simulink library "FirUp"  (R2022b)
settings: Solver=VariableStepAuto  StartTime=0.0  StopTime=10.0  RelTol=1e-3
undefined symbols (not defined in the file or in its folder): Row
libraries: HandyTextFile x10, FeaturePath x2, ITC x2, $bdroot x2, TuneVar x2, dspmlti4 x1, FirGeneric x1, TOP x1
settings Model: Creator=jb10849  LastModifiedBy=sc48041
settings SolverCC: AlgebraicLoopSolver=TrustRegion
settings DebuggingCC: UnconnectedInputMsg=warning  UnconnectedOutputMsg=warning  UnconnectedLineMsg=warning  SFMachineParentedDataDiag=warning  ArithmeticOperatorsInVariantConditions=warning
settings ModelReferenceCC: EnableRefExpFcnMdlSchedulingChecks=on
settings SFSimCC: SimUseLocalCustomCode=off  CustomCodeUndefinedFunction=UseInterfaceOnly
settings RTWCC: RTWUseLocalCustomCode=off  DLArmComputeVersion=19.05
settings CodeAppCC: StateflowObjectComments=on

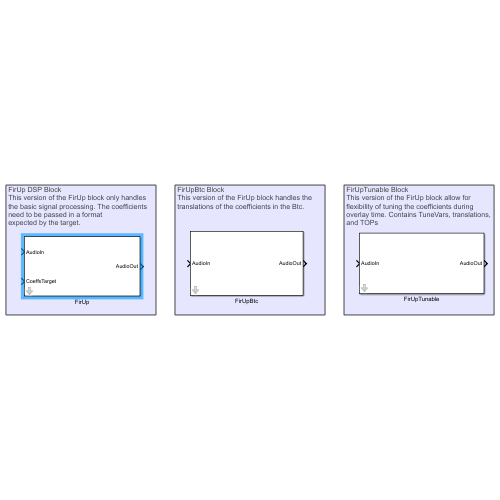
[thumbnail: Simulink's stored preview of the top-level diagram]
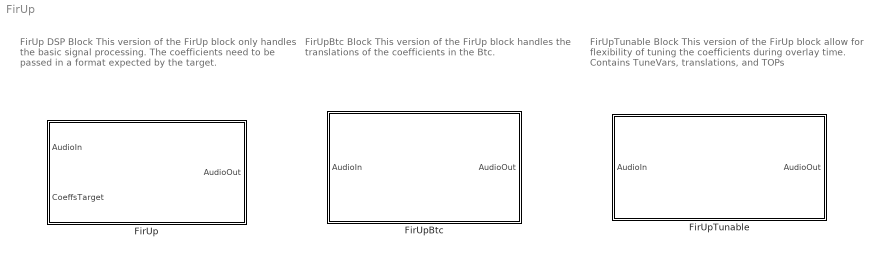
== system FirUp ==
  note: FirUp DSP Block
      | This version of the FirUp block only handles
      | the basic signal processing. The coefficients
      | need to be passed in a format
      | expected by the target.
  note: FirUpBtc Block
      | This version of the FirUp block handles the
      | translations of the coefficients in the Btc.
  note: FirUpTunable Block
      | This version of the FirUp block allow for
      | flexibility of tuning the coefficients during
      | overlay time. Contains TuneVars, translations,
      | and TOPs
  FirUp : Subsystem  mask(Blocklib FirUp){Config=[]}
      mask prompts: Config "FirUpConfig"
      mask init:
      | blkh=gcbh;
      | Config=BTConfig.Assert(blkh,Config);
      | 
      | Config.Validate();
      | Config.DoMaskInit(blkh);
      mask DialogControl ParamterGroupVar Prompt: Parameters
  FirUpBtc : Subsystem  mask(Blocklib FirUpBtc){Config=[]}
      mask prompts: Config "FirUpBtcConfig"
      mask init:
      | blkh=gcbh;
      | Config=BTConfig.Assert(blkh,Config);
      | 
      | Config.Validate();
      | Config.DoMaskInit(blkh);
  FirUpTunable : Subsystem  mask(Blocklib FirUpTunable){Config=[]}
      mask prompts: Config "FirUpTunableConfig"
      mask init:
      | blkh=gcbh;
      | Config=BTConfig.Assert(blkh,Config);
      | 
      | Config.Validate();
      | Config.DoMaskInit(blkh);

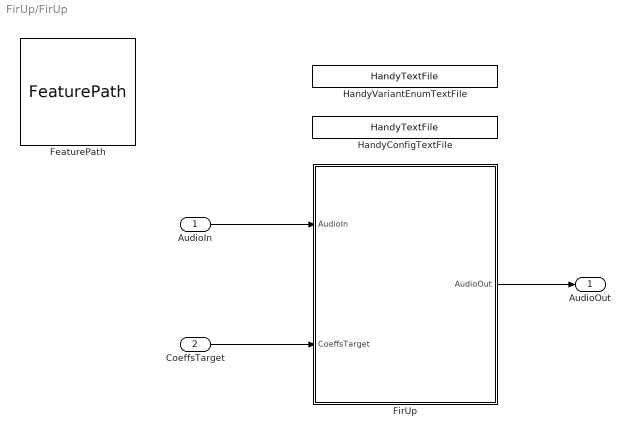
== system FirUp/FirUp ==
  AudioIn : Inport
  CoeffsTarget : Inport  Port=2
  FeaturePath : FeaturePath/FeaturePath  FeatureName=FirUp  IsGroup=off  GroupNumber=-1  IsModule=off  TriggerInit=[125 24 240 131]
      settings: SourceProductName=Bose Talaria
  FirUp : Subsystem  Variant=on
  HandyConfigTextFile : HandyTextFile/HandyTextFile  TemplateSource=Config  FileSuffix=File  OpenDialogOnLoad=off  UseThisBlockName=off  AddGrandParentNamePrefix=off  TheDefaultText=% $(FILENAME) $(PREFIX) $(SUFFIX)  ShowInLibBrowser=on
      settings: SourceProductName=Bose Talaria
  HandyVariantEnumTextFile : HandyTextFile/HandyTextFile  TemplateSource=VariantEnum  FileSuffix=File  OpenDialogOnLoad=off  UseThisBlockName=off  AddGrandParentNamePrefix=off  TheDefaultText=% $(FILENAME) $(PREFIX) $(SUFFIX)  ShowInLibBrowser=on
      settings: SourceProductName=Bose Talaria
  AudioOut : Outport
  wires:
  FirUp/1(AudioOut) -> AudioOut/1
  CoeffsTarget/1 -> FirUp/2(CoeffsTarget)
  AudioIn/1 -> FirUp/1(AudioIn)

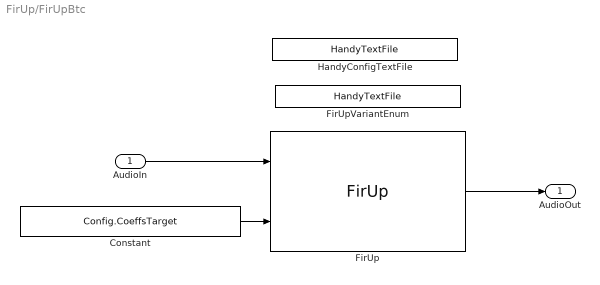
== system FirUp/FirUpBtc ==
  AudioIn : Inport
  Constant : Constant  Value=Config.CoeffsTarget  VectorParams1D=off  OutDataTypeStr=single
  FirUp : $bdroot/FirUp  Config=Config
  FirUpVariantEnum : HandyTextFile/HandyTextFile  TemplateSource=<dialog fields>  FileSuffix=VariantEnum  OpenDialogOnLoad=off  UseThisBlockName=on  AddGrandParentNamePrefix=off  TheDefaultText=% $(FILENAME) $(PREFIX) $(SUFFIX)  ShowInLibBrowser=on
      settings: SourceProductName=Bose Talaria
  HandyConfigTextFile : HandyTextFile/HandyTextFile  TemplateSource=Config  FileSuffix=File  OpenDialogOnLoad=off  UseThisBlockName=off  AddGrandParentNamePrefix=off  TheDefaultText=% $(FILENAME) $(PREFIX) $(SUFFIX)  ShowInLibBrowser=on
      settings: SourceProductName=Bose Talaria
  AudioOut : Outport
  wires:
  AudioIn/1 -> FirUp/1
  FirUp/1 -> AudioOut/1
  Constant/1 -> FirUp/2

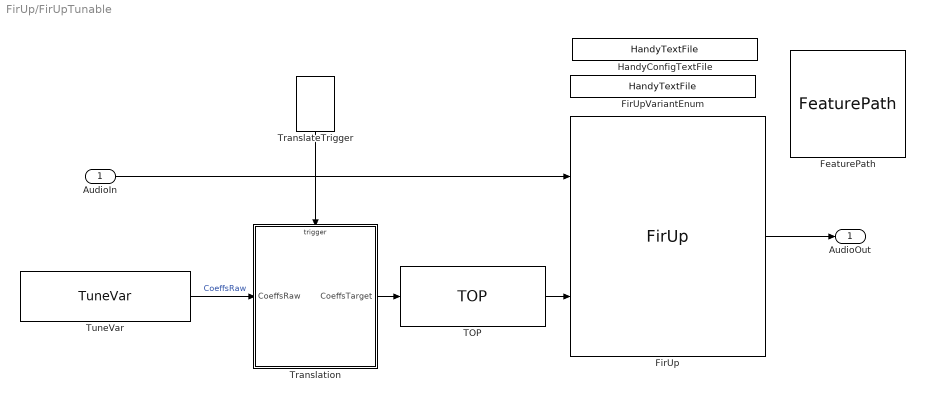
== system FirUp/FirUpTunable ==
  AudioIn : Inport
  FeaturePath : FeaturePath/FeaturePath  FeatureName=FirUp  IsGroup=off  GroupNumber=-1  IsModule=off  TriggerInit=[415 9 530 116]
      settings: SourceProductName=Bose Talaria
  FirUp : $bdroot/FirUp  Config=Config
  FirUpVariantEnum : HandyTextFile/HandyTextFile  TemplateSource=<dialog fields>  FileSuffix=File  OpenDialogOnLoad=off  UseThisBlockName=off  AddGrandParentNamePrefix=off  TheDefaultText=% $(FILENAME) $(PREFIX) $(SUFFIX)  ShowInLibBrowser=on
      settings: SourceProductName=Bose Talaria
  HandyConfigTextFile : HandyTextFile/HandyTextFile  TemplateSource=Config  FileSuffix=File  OpenDialogOnLoad=off  UseThisBlockName=off  AddGrandParentNamePrefix=off  TheDefaultText=% $(FILENAME) $(PREFIX) $(SUFFIX)  ShowInLibBrowser=on
      settings: SourceProductName=Bose Talaria
  TOP : TOP/TOP  TriggerInit=[25 225 170 285]  TopName=CoeffsTarget  DataTypeOut=Inherit: Same as input  BankNumber=0  PreOverlay=false  PostOverlay=false  Role=Automatic
      settings: SourceProductName=Bose Talaria
  TranslateTrigger : TuneVar/TranslateTrigger  TriggerInit=[-79 35 -41 90]
      settings: SourceProductName=Bose Talaria
  Translation : MATLAB Function  TreatAsAtomicUnit=on  mask(Talaria Translation){UpFactor=Config.UpFactor, VariantStr=Config.Variant.Uint8Str, WithFirVariantStr=Config.WithFirVariant.Uint8Str}
      mask help: This MATLAB Function Block can be automatically inserted by several automation routines. Once placed, the block is ready to accept translation logic from the model designer.
  TuneVar : TuneVar/TuneVar  TuneName=CoeffsRaw  SpecifyMaxSize=off  VariableDim=1 (Row)  MaxSize=[1 1]  TunabilityNumber=1  MinValue=[]  MaxValue=[]  TriggerInit=[-355 230 -185 280]  MaskValue=Config.TuneVarCoeffsRaw
      settings: SourceProductName=Bose Talaria
  AudioOut : Outport
  wires:
  FirUp/1 -> AudioOut/1
  AudioIn/1 -> FirUp/1
  TranslateTrigger/1 -> Translation/Trigger
  TuneVar/1 -> Translation/1(CoeffsRaw)  "CoeffsRaw"
  Translation/1(CoeffsTarget) -> TOP/1
  TOP/1 -> FirUp/2

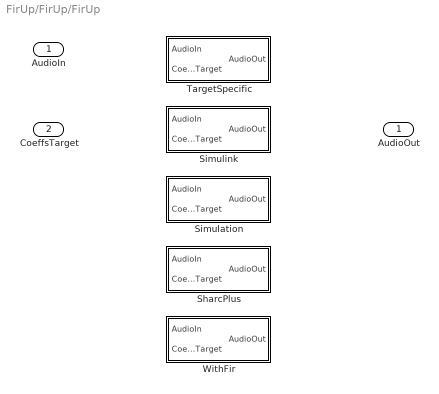
== system FirUp/FirUp/FirUp ==
  AudioIn : Inport
  CoeffsTarget : Inport  Port=2
  SharcPlus : Subsystem  VariantControl=Config.Variant.StartsWith('SharcPlus')
  Simulation : Subsystem  VariantControl=Config.Variant.StartsWith('Simulation')
  Simulink : Subsystem  VariantControl=(default)
  TargetSpecific : Subsystem  VariantControl=Config.Variant.StartsWith('Generic') || Config.Variant.StartsWith('Hexagon')
  WithFir : Subsystem  VariantControl=Config.Variant.StartsWith('WithFir')
  AudioOut : Outport

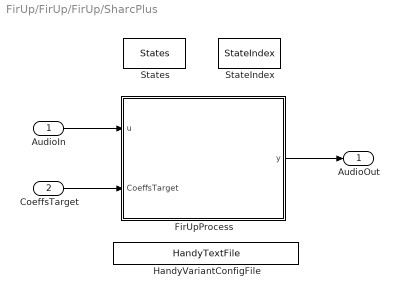
== system FirUp/FirUp/FirUp/SharcPlus ==
  AudioIn : Inport
  CoeffsTarget : Inport  Port=2
  FirUpProcess : MATLAB Function  TreatAsAtomicUnit=on  mask{UpFactor=Config.UpFactor}
  HandyVariantConfigFile : HandyTextFile/HandyTextFile  TemplateSource=VariantConfig  FileSuffix=Init  OpenDialogOnLoad=off  UseThisBlockName=off  AddGrandParentNamePrefix=on  TheDefaultText=|  ShowInLibBrowser=on
      | % $(FILENAME) Setup model parameters for each "Init" callback (e.g. update diagram)
      | sample_rate_in_hertz = 44100;
      | frame_size = 32;
      | sysin_channel_count = 2;
      settings: SourceProductName=Bose Talaria
  StateIndex : DataStoreMemory  DataStoreName=StateIndex  InitialValue=Config.VariantObj.DsmStateIndexInitValue  ShowAdditionalParam=off  OutDataTypeStr=int32
  States : DataStoreMemory  DataStoreName=States  InitialValue=Config.VariantObj.DsmStatesInitValue  ShowAdditionalParam=off  OutDataTypeStr=single
  AudioOut : Outport
  wires:
  FirUpProcess/1(y) -> AudioOut/1
  AudioIn/1 -> FirUpProcess/1(u)
  CoeffsTarget/1 -> FirUpProcess/2(CoeffsTarget)

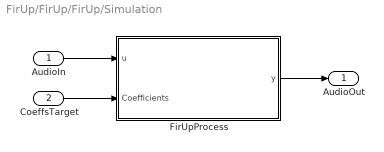
== system FirUp/FirUp/FirUp/Simulation ==
  AudioIn : Inport
  CoeffsTarget : Inport  Port=2
  FirUpProcess : MATLAB Function  TreatAsAtomicUnit=on  mask{UpFactor=Config.UpFactor}
  AudioOut : Outport
  wires:
  AudioIn/1 -> FirUpProcess/1(u)
  FirUpProcess/1(y) -> AudioOut/1
  CoeffsTarget/1 -> FirUpProcess/2(Coefficients)

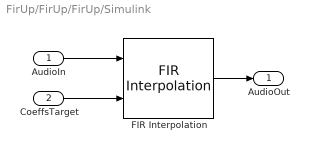
== system FirUp/FirUp/FirUp/Simulink ==
  AudioIn : Inport  OutDataTypeStr=single
  CoeffsTarget : Inport  Port=2  OutDataTypeStr=single
  FIR Interpolation : dspmlti4/FIR Interpolation  FilterSource=Input port  PrivateCoeffs=0  h=Config.Coefficients  L=Config.UpFactor  FilterObject=FINTERP  InputProcessing=Columns as channels (frame based)  framing=Enforce single-rate processing  outputBufInitCond=0  roundingMode=Floor  overflowMode=off  firstCoeffDataTypeStr=Inherit: Same word length as input  firstCoeffMin=[]  firstCoeffMax=[]  firstCoeffLastDataTypeStr=Inherit: Same word length as input  outputDataTypeStr=Inherit: Same as accumulator  outputMin=[]  outputMax=[]  outputLastDataTypeStr=Inherit: Same as accumulator
  AudioOut : Outport  OutDataTypeStr=single
  wires:
  AudioIn/1 -> FIR Interpolation/1
  FIR Interpolation/1 -> AudioOut/1
  CoeffsTarget/1 -> FIR Interpolation/2

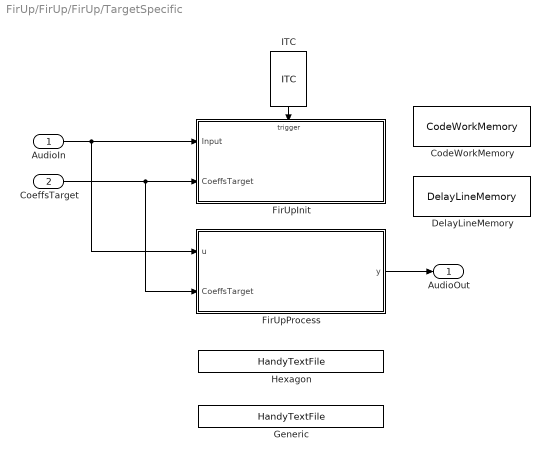
== system FirUp/FirUp/FirUp/TargetSpecific ==
  AudioIn : Inport
  CoeffsTarget : Inport  Port=2
  CodeWorkMemory : DataStoreMemory  DataStoreName=CodeWorkMemory  WriteAfterWriteMsg=warning  InitialValue=Config.VariantObj.CodeWorkMemoryInitValue  ShowAdditionalParam=off  OutDataTypeStr=uint32
  DelayLineMemory : DataStoreMemory  DataStoreName=DelayLineMemory  WriteAfterWriteMsg=warning  InitialValue=Config.VariantObj.DelayLineMemoryInitValue  ShowAdditionalParam=off  OutDataTypeStr=single
  FirUpInit : MATLAB Function  TreatAsAtomicUnit=on  mask{UpFactor=Config.UpFactor, VariantUint8=Config.Variant.Uint8Str}
  FirUpProcess : MATLAB Function  TreatAsAtomicUnit=on  mask{UpFactor=Config.UpFactor, VariantUint8=Config.Variant.Uint8Str}
  Generic : HandyTextFile/HandyTextFile  TemplateSource=VariantConfig  FileSuffix=Init  OpenDialogOnLoad=off  UseThisBlockName=on  AddGrandParentNamePrefix=on  TheDefaultText=|  ShowInLibBrowser=on
      | % $(FILENAME) Setup model parameters for each "Init" callback (e.g. update diagram)
      | sample_rate_in_hertz = 44100;
      | frame_size = 32;
      | sysin_channel_count = 2;
      settings: SourceProductName=Bose Talaria
  Hexagon : HandyTextFile/HandyTextFile  TemplateSource=VariantConfig  FileSuffix=Init  OpenDialogOnLoad=off  UseThisBlockName=on  AddGrandParentNamePrefix=on  TheDefaultText=|  ShowInLibBrowser=on
      | % $(FILENAME) Setup model parameters for each "Init" callback (e.g. update diagram)
      | sample_rate_in_hertz = 44100;
      | frame_size = 32;
      | sysin_channel_count = 2;
      settings: SourceProductName=Bose Talaria
  ITC : ITC/ITC
      settings: SourceProductName=Bose Talaria
  AudioOut : Outport
  wires:
  FirUpProcess/1(y) -> AudioOut/1
  ITC/1 -> FirUpInit/Trigger
  AudioIn/1 -> FirUpProcess/1(u), FirUpInit/1(Input)
  CoeffsTarget/1 -> FirUpProcess/2(CoeffsTarget), FirUpInit/2(CoeffsTarget)

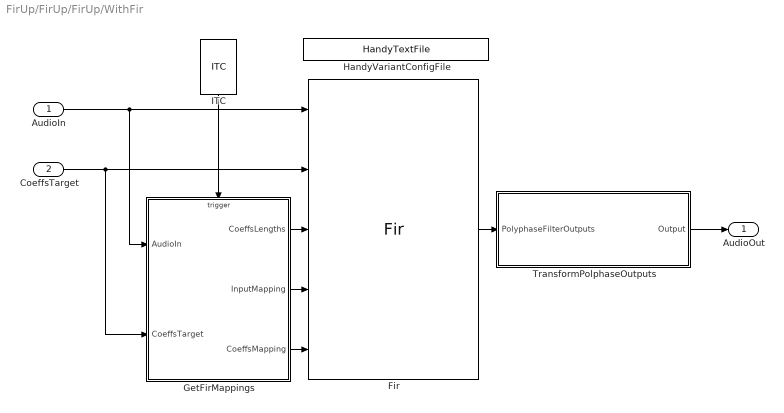
== system FirUp/FirUp/FirUp/WithFir ==
  AudioIn : Inport
  CoeffsTarget : Inport  Port=2
  Fir : FirGeneric/Fir  Config=Config.VariantObj.Fir
      settings: SourceProductName=Bose Blocklib
  GetFirMappings : MATLAB Function  TreatAsAtomicUnit=on  mask{UpFactor=Config.UpFactor}
  HandyVariantConfigFile : HandyTextFile/HandyTextFile  TemplateSource=VariantConfig  FileSuffix=Init  OpenDialogOnLoad=off  UseThisBlockName=off  AddGrandParentNamePrefix=on  TheDefaultText=|  ShowInLibBrowser=on
      | % $(FILENAME) Setup model parameters for each "Init" callback (e.g. update diagram)
      | sample_rate_in_hertz = 44100;
      | frame_size = 32;
      | sysin_channel_count = 2;
      settings: SourceProductName=Bose Talaria
  ITC : ITC/ITC
      settings: SourceProductName=Bose Talaria
  TransformPolphaseOutputs : MATLAB Function  TreatAsAtomicUnit=on  mask{UpFactor=Config.UpFactor}
  AudioOut : Outport
  wires:
  GetFirMappings/1(CoeffsLengths) -> Fir/3
  GetFirMappings/3(CoeffsMapping) -> Fir/5
  GetFirMappings/2(InputMapping) -> Fir/4
  ITC/1 -> GetFirMappings/Trigger
  TransformPolphaseOutputs/1(Output) -> AudioOut/1
  CoeffsTarget/1 -> GetFirMappings/2(CoeffsTarget), Fir/2
  Fir/1 -> TransformPolphaseOutputs/1(PolyphaseFilterOutputs)
  AudioIn/1 -> GetFirMappings/1(AudioIn), Fir/1

== matlab function FirUp/FirUp/TargetSpecific/FirUpProcess ==
  data: u input; y output; UpFactor parameter; DelayLineMemory data_store_memory; CodeWorkMemory data_store_memory; VariantUint8 parameter; CoeffsTarget input
function y = FirUpProcess(u, UpFactor, VariantUint8, CoeffsTarget)
% Upsample the input signal by an integer-valued factor, then apply an 
% FIR filter. 

global DelayLineMemory;
global CodeWorkMemory;
VariantSelect = char(VariantUint8);

if(coder.target('MATLAB') || coder.target('Sfun')) 
    y = FirUpProcessSim(u, CoeffsTarget, UpFactor, VariantSelect);
else
    switch(VariantSelect)
        case('Generic')
            y = firup_generic_process(single(u), single(DelayLineMemory), uint32(CodeWorkMemory), uint32(UpFactor));
        case('Hexagon')
            y = firup_hexagon_process(single(u), single(DelayLineMemory), uint32(CodeWorkMemory), uint32(UpFactor));
    end
end
end

function y = firup_generic_process(u, DelayLineMemory, CodeWorkMemory, UpFactor)
coder.replace('-errorifnoreplacement');
[FrameSize, NumChannels] = size(u);
y = single(zeros(FrameSize*UpFactor, NumChannels));
end
function y = firup_hexagon_process(u, DelayLineMemory, CodeWorkMemory, UpFactor)
coder.replace('-errorifnoreplacement');
[FrameSize, NumChannels] = size(u);
y = single(zeros(FrameSize*UpFactor, NumChannels));
end

== matlab function FirUp/FirUp/SharcPlus/FirUpProcess ==
  data: u input; CoeffsTarget input; y output; UpFactor parameter; States data_store_memory; StateIndex data_store_memory
function y = FirUpProcess(u, CoeffsTarget, UpFactor)
% Upsample the input signal by an integer-valued factor, then apply an 
% FIR filter. 
global States;
global StateIndex;

if(coder.target('MATLAB') || coder.target('Sfun')) 
    y = FirUpProcessSim(u, CoeffsTarget, UpFactor, "SharcPlus");
else
    [FrameSize, NumChannels] = size(u);
    ActiveCoeffSet = zeros(NumChannels,1);
    PolyphaseFilterLength = numel(CoeffsTarget)/ UpFactor;
    y = upfir(single(u), uint32(FrameSize*UpFactor), uint32(NumChannels), single(States), ...
        int32(numel(CoeffsTarget)), int32(StateIndex), single(CoeffsTarget), ...
        uint32(ActiveCoeffSet), int32(UpFactor), int32(PolyphaseFilterLength));
end
end

function y = upfir(u, framesize, numChannels, states2, filterLength, stateIndex2, coeffs, activeCoeffSet, interp_factor, polylen)
% If target == codegen, generate warning if no CRL found
coder.replace('-errorifnoreplacement');
y = single(zeros(framesize , numChannels));
end

== matlab function FirUp/FirUp/TargetSpecific/FirUpInit ==
  data: Input input; UpFactor parameter; CodeWorkMemory data_store_memory; VariantUint8 parameter; CoeffsTarget input
  events: trigger input FUNCTION_CALL_EVENT
function FirUpInit(Input, UpFactor, VariantUint8, CoeffsTarget)

global CodeWorkMemory;

VariantSelect = char(VariantUint8);
[FrameSize, NumChannels] = size(Input);
FilterLength = numel(CoeffsTarget);
if(coder.target('MATLAB') || coder.target('Sfun')) 
    return;
else
    switch(VariantSelect)
        case('Generic')
            y = firup_generic_init(single(CoeffsTarget), uint32(FrameSize), uint32(UpFactor), uint32(FilterLength), uint32(NumChannels), uint32(CodeWorkMemory));
            % NOTE: The CRL mechanism requires an output for the function call,
            % and appears to be optimized out if that return value isn't used. 
            % This is a dummy operation to make sure CRL ends up in generated code
            CodeWorkMemory(1) = y;
        case('Hexagon')
            y = firup_hexagon_init(single(CoeffsTarget), uint32(FrameSize), uint32(UpFactor), uint32(FilterLength), uint32(NumChannels), uint32(CodeWorkMemory));
            % NOTE: The CRL mechanism requires an output for the function call,
            % and appears to be optimized out if that return value isn't used. 
            % This is a dummy operation to make sure CRL ends up in generated code
            CodeWorkMemory(1) = y;
    end
end
end

function y = firup_generic_init(CoeffsTarget, FrameSize, UpFactor, FilterLength, NumChannels, CodeWorkMemory)
coder.replace('-warnifnoreplacement');
y = CodeWorkMemory(1) + 1;
end
function y = firup_hexagon_init(CoeffsTarget, FrameSize, UpFactor, FilterLength, NumChannels, CodeWorkMemory)
coder.replace('-errorifnoreplacement');
y = CodeWorkMemory(1) + 1;
end

== matlab function FirUp/FirUp/Simulation/FirUpProcess ==
  data: u input; y output; UpFactor parameter; Coefficients input
function y = FirUpProcess(u, UpFactor, Coefficients)
% Upsample the input signal by an integer-valued factor, then apply an 
% FIR filter. 
y = FirUpProcessSim(u, Coefficients, UpFactor);
end

== matlab function FirUp/FirUp/WithFir/GetFirMappings ==
  data: AudioIn input; CoeffsTarget input; CoeffsLengths output; InputMapping output; CoeffsMapping output; UpFactor parameter
  events: trigger input FUNCTION_CALL_EVENT
function [CoeffsLengths, InputMapping, CoeffsMapping] = GetFirMappings(AudioIn, CoeffsTarget, UpFactor)

[~, NumChannels] = size(AudioIn);
NumOutputs = UpFactor*NumChannels;

% Coefficients are equally divided up into [UpFactor] number of coefficient
% sets. 
% CoeffsLengths = uint32(ceil(ones(1,UpFactor).*(numel(CoeffsTarget)/UpFactor)));
CoeffsLengths = uint32(ceil(ones(1,NumOutputs).*(numel(CoeffsTarget)/UpFactor)));


% Output is mapped as follows, where UpFactor = L and NumChannels = Nc
% ix = 0: Nc - 1
%   iy = 0: L - 1
% fcn(Input[ix], Filter[iy]) = Output[ix*L + iy]
%
% CoeffsMapping = [0, 1, 2 ... L-1, 0, 1, 2 ... L-1 ...]
CoeffsMapping = uint32(mod(0:NumOutputs-1,UpFactor));
% InputMapping = [0 0 0 0 ... 1 1 1 1 ... 2 2 2 2 ... Nc-1 Nc-1 Nc-1 Nc-1 ...]
InputMapping = uint32(reshape(repmat(0:NumChannels-1,UpFactor,1),1,[])');

end

== matlab function FirUp/FirUp/WithFir/TransformPolphaseOutputs ==
  data: PolyphaseFilterOutputs input; Output output; UpFactor parameter
function Output = TransformPolyphaseOutputs(PolyphaseFilterOutputs, UpFactor)
% Converts polyphase filter outputs into standard filter outputs

% Instantiate output array
[FrameSizeIn, PolyphaseChannels] = size(PolyphaseFilterOutputs);
NumChannels = PolyphaseChannels/UpFactor;
Output = zeros(FrameSizeIn*UpFactor, PolyphaseChannels/UpFactor,'single');
for ch = 1: NumChannels
    % Commutation of polyphase subfilter outputs into a single upsampled
    % output
    Output(:,ch) = reshape(PolyphaseFilterOutputs(:,(ch-1)*UpFactor + (1:UpFactor))',1,[]);
end
end

== matlab function FirUp/FirUpTunable/Translation ==
  data: CoeffsTarget output; CoeffsRaw input; UpFactor parameter; VariantStr parameter; WithFirVariantStr parameter
  events: trigger input FUNCTION_CALL_EVENT
function CoeffsTarget  = fcn(CoeffsRaw, UpFactor, VariantStr, WithFirVariantStr)
%#codegen

% ----- To access TuneVar maximum size, current size, and current value:
%   Note: TuneVar signals arrive with exposed variable size information.
%         The expressions below illustrate for the "Tune1" input argument.
%
%   size(Tune1.Value) : the maximum possible size of the Tune1 variable
%
%   Tune.Size   : the current size of *valid* data in Tune1.Value
%
%   Tune1.Size(1) : Number of rows present in Tune1 - this does not vary.
%
%   Tune1.Size(2) : Number of columns currently valid in Tune1 - this is
%       the variable part of size that can change (if allowed by TuneVar).
%
%   Tune1.Value : the current value of the tune variable... but end-padded 
%       to the maximum available size with undefined/invalid data.
%
%   numel(Tune1.Value) : another way of looking at the maximum number of
%       elements that could arrive in Tune1.Value
%
% ----- To register an error, use the following method (works like printf):
%   TranslateError( <format string>, <arguments ... )
%   ... this error will cause the build process to abort.
% ----- For warnings (works like printf):
%   TranslateWarning( <format string>, <arguments ... )
%   ... this warning will not set the translation engine error state.

% Convert VariantEnum type to string
Variant = char(VariantStr);
WithFirVariantStr = char(WithFirVariantStr);
% Set default value if arg not specified
CoeffsTarget = FirUpTranslation(CoeffsRaw.Value, UpFactor, Variant, WithFirVariantStr);

end
